simulink model "ALL_JP360_DBW_V6_5_1103"  (R2022a)
settings: Solver=FixedStepAuto  StartTime=0.0  StopTime=inf  FixedStep=0.01  RelTol=1e-3  EnableMultiTasking=on
model workspace (MAT data in the model file):
  g = 9.8
undefined symbols (not defined in the file or in its folder): canChannel, delta_v_p, IPM_Line_C0, IPM_Line_C1, IPM_Line_C2, IPM_Line_C3, M, M_p, MRR_ObjDistX, MRR_ObjDistY, MRR_ObjFusionCamID, MRR_ObjFusionSig, MRR_ObjID, MRR_ObjRelVelX, MRR_ObjRelVelY, MRR_ObjType, MRR_ObjUpdFlg, none, obj_vaild, untracktime, V, videoinput
libraries: canfdmsglib x230, canfdlib x76, slpidlib x24, simulink x18, dspstat3 x14, ctrlSharedLib x1, simulink_extras x1, imaqlib x1, realtime_pacer_lib x1, dspvision x1, visionsinks x1
(part 14 of 55)

== system ALL_JP360_DBW_V6_5_1103/MsgFromCAN/CCAN_GW_MsgFromCAN/CCAN_GW_GW_ESP_CCO_0x252 ==
  CCAN_GW_GW_ESP_CCO_0x252FromInData : Inport  OutDataTypeStr=Bus:CAN_FD_MESSAGE_BUS
  Bus Creator : BusCreator  Inputs=9  OutDataTypeStr=Bus:CCAN_GW_GW_ESP_CCO_0x252  NonVirtualBus=on
  CAN FD Unpack : canfdmsglib/CAN FD Unpack  CANdbFile=HiFire_JPT360_CCAN_Matrix_CAN_V1.72_VP_ADCU.dbc  MsgList=(none)  MsgName=GW_ESP_CCO_0x252  ProtocolMode=CAN FD  MsgIDType=Standard (11-bit identifier)  MsgIdentifier=594  MsgLength=8  SignalInfo={'Checksum_0x252','56','8','BE','unsigned','Standard','0','1','0','0','255';'ESP_CCOSts','6','2','BE','unsigned','Standard','0','1','0','0','3';'ESP_CCOTgtVel','14','5','BE','unsigned','Standard','0','1','0','0','30';'ESP_CCOWarning_Message','3','3','BE','unsigned','Standard','0','1','0','0','4';'ESP_CCO_Torque_Request','24','16','BE','unsigned','Standard','0','1','-30000','-30000','30000';'ESP_CCO_Torque_Request_Status','13','1','BE','unsigned','Standard','0','1','0','0','1';'ESP_TABSts','11','2','BE','unsigned','Standard','0','1','0','0','3';'ESP_TABWarning_Message','9','2','BE','unsigned','Standard','0','1','0','0','3';'RollingCounter_0x252','48','4','BE','unsigned','Standard','0','1','0','0','15'}  IDPort=off  TimestampPort=off  ErrorPort=off  RemotePort=off  LengthPort=off  StatusPort=off  BRSPort=off  ESIPort=off  DLCPort=off  ApplyMinMax=off
      settings: SourceProductBaseCode=XP,ME,VN  DataFormat=CANdb specified signals
  Data Type Conversion1 : DataTypeConversion  OutDataTypeStr=uint8  SaturateOnIntegerOverflow=off  RndMeth=Floor
  Data Type Conversion{2..4,7..9} (6 alike) : DataTypeConversion  OutDataTypeStr=int8  SaturateOnIntegerOverflow=off  RndMeth=Floor
  Data Type Conversion5 : DataTypeConversion  OutDataTypeStr=int16  SaturateOnIntegerOverflow=off  RndMeth=Floor
  Data Type Conversion6 : DataTypeConversion  OutDataTypeStr=boolean  SaturateOnIntegerOverflow=off  RndMeth=Floor
  CCAN_GW_GW_ESP_CCO_0x252FromOutData : Outport  OutDataTypeStr=Bus:CCAN_GW_GW_ESP_CCO_0x252
  wires:
  CAN FD Unpack/1 -> Data Type Conversion1/1
  CAN FD Unpack/2 -> Data Type Conversion2/1
  CAN FD Unpack/3 -> Data Type Conversion3/1
  CAN FD Unpack/4 -> Data Type Conversion4/1
  CAN FD Unpack/5 -> Data Type Conversion5/1
  CAN FD Unpack/6 -> Data Type Conversion6/1
  CAN FD Unpack/7 -> Data Type Conversion7/1
  CAN FD Unpack/8 -> Data Type Conversion8/1
  CAN FD Unpack/9 -> Data Type Conversion9/1
  Data Type Conversion1/1 -> Bus Creator/1  "Checksum_0x252"
  Data Type Conversion2/1 -> Bus Creator/2  "ESP_CCOSts"
  Data Type Conversion3/1 -> Bus Creator/3  "ESP_CCOTgtVel"
  Data Type Conversion4/1 -> Bus Creator/4  "ESP_CCOWarning_Message"
  Data Type Conversion5/1 -> Bus Creator/5  "ESP_CCO_Torque_Request"
  Data Type Conversion6/1 -> Bus Creator/6  "ESP_CCO_Torque_Request_Status"
  Data Type Conversion7/1 -> Bus Creator/7  "ESP_TABSts"
  Data Type Conversion8/1 -> Bus Creator/8  "ESP_TABWarning_Message"
  Data Type Conversion9/1 -> Bus Creator/9  "RollingCounter_0x252"
  Bus Creator/1 -> CCAN_GW_GW_ESP_CCO_0x252FromOutData/1  "CCAN_GW_GW_ESP_CCO_0x252FromOutData"
  CCAN_GW_GW_ESP_CCO_0x252FromInData/1 -> CAN FD Unpack/1  "CCAN_GW_GW_ESP_CCO_0x252FromInData"

== system ALL_JP360_DBW_V6_5_1103/MsgFromCAN/CCAN_GW_MsgFromCAN/CCAN_GW_IPM_0x245 ==
  CCAN_GW_IPM_0x245FromInData : Inport  OutDataTypeStr=Bus:CAN_FD_MESSAGE_BUS
  Bus Creator : BusCreator  Inputs=21  OutDataTypeStr=Bus:CCAN_GW_IPM_0x245  NonVirtualBus=on
  CAN FD Unpack : canfdmsglib/CAN FD Unpack  CANdbFile=HiFire_JPT360_CCAN_Matrix_CAN_V1.72_VP_ADCU.dbc  MsgList=(none)  MsgName=IPM_0x245  ProtocolMode=CAN FD  MsgIDType=Standard (11-bit identifier)  MsgIdentifier=581  MsgLength=8  SignalInfo={'Checksum_0x245','56','8','BE','unsigned','Standard','0','1','0','0','255';'IPM_ADAS_Alerts','43','3','BE','unsigned','Standard','0','1','0','0','7';'IPM_IHC_HighbeamReq','55','1','BE','unsigned','Standard','0','1','0','0','1';'IPM_IHC_Status','40','3','BE','unsigned','Standard','0','1','0','0','7';'IPM_LDWWarningType','52','2','BE','unsigned','Standard','0','1','0','0','3';'IPM_LaneAssitType','22','3','BE','unsigned','Standard','0','1','0','0','7';'IPM_LaneAssit_HandsonReq','54','1','BE','unsigned','Standard','0','1','0','0','1';'IPM_LaneAssit_LeftVisualization','18','2','BE','unsigned','Standard','0','1','0','0','3';'IPM_LaneAssit_RightVisualization','20','2','BE','unsigned','Standard','0','1','0','0','3';'IPM_LaneAssit_Sensitivity','16','1','BE','unsigned','Standard','0','1','0','0','1';'IPM_LaneAssit_Status','29','3','BE','unsigned','Standard','0','1','0','0','7';'IPM_LaneAssit_TorqueReq','13','11','BE','unsigned','Standard','0','0.01','-10.24','-10.24','10.22';'IPM_LaneAssit_TorqueReqStatus','10','2','BE','unsigned','Standard','0','1','0','0','3';'IPM_LaneAssit_TorqueValidity','12','1','BE','unsigned','Standard','0','1','0','0','1';'IPM_LaneAssit_WarningAudio','17','1','BE','unsigned','Standard','0','1','0','0','1';'IPM_LaneAssit_WarningVibration','9','1','BE','unsigned','Standard','0','1','0','0','1';'IPM_SLA_Spdlimit','32','8','BE','unsigned','Standard','0','1','0','0','255';'IPM_SLA_SpdlimitUnits','24','2','BE','unsigned','Standard','0','1','0','0','3';'IPM_SLA_Status','26','3','BE','unsigned','Standard','0','1','0','0','7';'IPM_TJAICA_Status','47','1','BE','unsigned','Standard','0','1','0','0','1';'RollingCounter_0x245','48','4','BE','unsigned','Standard','0','1','0','0','15'}  IDPort=off  TimestampPort=off  ErrorPort=off  RemotePort=off  LengthPort=off  StatusPort=off  BRSPort=off  ESIPort=off  DLCPort=off  ApplyMinMax=off
      settings: SourceProductBaseCode=XP,ME,VN  DataFormat=CANdb specified signals
  Data Type Conversion1 : DataTypeConversion  OutDataTypeStr=uint8  SaturateOnIntegerOverflow=off  RndMeth=Floor
  Data Type Conversion{3,7,10,14..16,20} (7 alike) : DataTypeConversion  OutDataTypeStr=boolean  SaturateOnIntegerOverflow=off  RndMeth=Floor
  Data Type Conversion{2,4..6,8..9,11,13,18..19,21} (11 alike) : DataTypeConversion  OutDataTypeStr=int8  SaturateOnIntegerOverflow=off  RndMeth=Floor
  Data Type Conversion12 : DataTypeConversion  OutDataTypeStr=single  SaturateOnIntegerOverflow=off  RndMeth=Floor
  Data Type Conversion17 : DataTypeConversion  OutDataTypeStr=uint8  SaturateOnIntegerOverflow=off  RndMeth=Floor
  CCAN_GW_IPM_0x245FromOutData : Outport  OutDataTypeStr=Bus:CCAN_GW_IPM_0x245
  wires:
  CAN FD Unpack/1 -> Data Type Conversion1/1
  CAN FD Unpack/2 -> Data Type Conversion2/1
  CAN FD Unpack/3 -> Data Type Conversion3/1
  CAN FD Unpack/4 -> Data Type Conversion4/1
  CAN FD Unpack/5 -> Data Type Conversion5/1
  CAN FD Unpack/6 -> Data Type Conversion6/1
  CAN FD Unpack/7 -> Data Type Conversion7/1
  CAN FD Unpack/8 -> Data Type Conversion8/1
  CAN FD Unpack/9 -> Data Type Conversion9/1
  CAN FD Unpack/10 -> Data Type Conversion10/1
  CAN FD Unpack/11 -> Data Type Conversion11/1
  CAN FD Unpack/12 -> Data Type Conversion12/1
  CAN FD Unpack/13 -> Data Type Conversion13/1
  CAN FD Unpack/14 -> Data Type Conversion14/1
  CAN FD Unpack/15 -> Data Type Conversion15/1
  CAN FD Unpack/16 -> Data Type Conversion16/1
  CAN FD Unpack/17 -> Data Type Conversion17/1
  CAN FD Unpack/18 -> Data Type Conversion18/1
  CAN FD Unpack/19 -> Data Type Conversion19/1
  CAN FD Unpack/20 -> Data Type Conversion20/1
  CAN FD Unpack/21 -> Data Type Conversion21/1
  Data Type Conversion1/1 -> Bus Creator/1  "Checksum_0x245"
  Data Type Conversion2/1 -> Bus Creator/2  "IPM_ADAS_Alerts"
  Data Type Conversion3/1 -> Bus Creator/3  "IPM_IHC_HighbeamReq"
  Data Type Conversion4/1 -> Bus Creator/4  "IPM_IHC_Status"
  Data Type Conversion5/1 -> Bus Creator/5  "IPM_LDWWarningType"
  Data Type Conversion6/1 -> Bus Creator/6  "IPM_LaneAssitType"
  Data Type Conversion7/1 -> Bus Creator/7  "IPM_LaneAssit_HandsonReq"
  Data Type Conversion8/1 -> Bus Creator/8  "IPM_LaneAssit_LeftVisualization"
  Data Type Conversion9/1 -> Bus Creator/9  "IPM_LaneAssit_RightVisualization"
  Data Type Conversion10/1 -> Bus Creator/10  "IPM_LaneAssit_Sensitivity"
  Data Type Conversion11/1 -> Bus Creator/11  "IPM_LaneAssit_Status"
  Data Type Conversion12/1 -> Bus Creator/12  "IPM_LaneAssit_TorqueReq"
  Data Type Conversion13/1 -> Bus Creator/13  "IPM_LaneAssit_TorqueReqStatus"
  Data Type Conversion14/1 -> Bus Creator/14  "IPM_LaneAssit_TorqueValidity"
  Data Type Conversion15/1 -> Bus Creator/15  "IPM_LaneAssit_WarningAudio"
  Data Type Conversion16/1 -> Bus Creator/16  "IPM_LaneAssit_WarningVibration"
  Data Type Conversion17/1 -> Bus Creator/17  "IPM_SLA_Spdlimit"
  Data Type Conversion18/1 -> Bus Creator/18  "IPM_SLA_SpdlimitUnits"
  Data Type Conversion19/1 -> Bus Creator/19  "IPM_SLA_Status"
  Data Type Conversion20/1 -> Bus Creator/20  "IPM_TJAICA_Status"
  Data Type Conversion21/1 -> Bus Creator/21  "RollingCounter_0x245"
  Bus Creator/1 -> CCAN_GW_IPM_0x245FromOutData/1  "CCAN_GW_IPM_0x245FromOutData"
  CCAN_GW_IPM_0x245FromInData/1 -> CAN FD Unpack/1  "CCAN_GW_IPM_0x245FromInData"

== system ALL_JP360_DBW_V6_5_1103/MsgFromCAN/CCAN_GW_MsgFromCAN/CCAN_GW_IPM_0x247 ==
  CCAN_GW_IPM_0x247FromInData : Inport  OutDataTypeStr=Bus:CAN_FD_MESSAGE_BUS
  Bus Creator : BusCreator  Inputs=7  OutDataTypeStr=Bus:CCAN_GW_IPM_0x247  NonVirtualBus=on
  CAN FD Unpack : canfdmsglib/CAN FD Unpack  CANdbFile=HiFire_JPT360_CCAN_Matrix_CAN_V1.72_VP_ADCU.dbc  MsgList=(none)  MsgName=IPM_0x247  ProtocolMode=CAN FD  MsgIDType=Standard (11-bit identifier)  MsgIdentifier=583  MsgLength=8  SignalInfo={'Checksum_0x247','56','8','BE','unsigned','Standard','0','1','0','0','255';'IPM_DCLCSts','5','3','BE','unsigned','Standard','0','1','0','0','7';'IPM_DCLC_manualfeedback','14','4','BE','unsigned','Standard','0','1','0','0','15';'IPM_ELKSts','2','3','BE','unsigned','Standard','0','1','0','0','7';'IPM_Traffic_Sign_Dis','16','8','BE','unsigned','Standard','0','1','0','0','255';'IPM_TurnIndicatorReq','12','2','BE','unsigned','Standard','0','1','0','0','3';'RollingCounter_0x247','48','4','BE','unsigned','Standard','0','1','0','0','15'}  IDPort=off  TimestampPort=off  ErrorPort=off  RemotePort=off  LengthPort=off  StatusPort=off  BRSPort=off  ESIPort=off  DLCPort=off  ApplyMinMax=off
      settings: SourceProductBaseCode=XP,ME,VN  DataFormat=CANdb specified signals
  Data Type Conversion1 : DataTypeConversion  OutDataTypeStr=uint8  SaturateOnIntegerOverflow=off  RndMeth=Floor
  Data Type Conversion{2..4,6..7} (5 alike) : DataTypeConversion  OutDataTypeStr=int8  SaturateOnIntegerOverflow=off  RndMeth=Floor
  Data Type Conversion5 : DataTypeConversion  OutDataTypeStr=uint8  SaturateOnIntegerOverflow=off  RndMeth=Floor
  CCAN_GW_IPM_0x247FromOutData : Outport  OutDataTypeStr=Bus:CCAN_GW_IPM_0x247
  wires:
  CAN FD Unpack/1 -> Data Type Conversion1/1
  CAN FD Unpack/2 -> Data Type Conversion2/1
  CAN FD Unpack/3 -> Data Type Conversion3/1
  CAN FD Unpack/4 -> Data Type Conversion4/1
  CAN FD Unpack/5 -> Data Type Conversion5/1
  CAN FD Unpack/6 -> Data Type Conversion6/1
  CAN FD Unpack/7 -> Data Type Conversion7/1
  Data Type Conversion1/1 -> Bus Creator/1  "Checksum_0x247"
  Data Type Conversion2/1 -> Bus Creator/2  "IPM_DCLCSts"
  Data Type Conversion3/1 -> Bus Creator/3  "IPM_DCLC_manualfeedback"
  Data Type Conversion4/1 -> Bus Creator/4  "IPM_ELKSts"
  Data Type Conversion5/1 -> Bus Creator/5  "IPM_Traffic_Sign_Dis"
  Data Type Conversion6/1 -> Bus Creator/6  "IPM_TurnIndicatorReq"
  Data Type Conversion7/1 -> Bus Creator/7  "RollingCounter_0x247"
  Bus Creator/1 -> CCAN_GW_IPM_0x247FromOutData/1  "CCAN_GW_IPM_0x247FromOutData"
  CCAN_GW_IPM_0x247FromInData/1 -> CAN FD Unpack/1  "CCAN_GW_IPM_0x247FromInData"

== system ALL_JP360_DBW_V6_5_1103/MsgFromCAN/CCAN_GW_MsgFromCAN/CCAN_GW_IPM_LeftLine_0x278 ==
  CCAN_GW_IPM_LeftLine_0x278FromInData : Inport  OutDataTypeStr=Bus:CAN_FD_MESSAGE_BUS
  Bus Creator : BusCreator  Inputs=6  OutDataTypeStr=Bus:CCAN_GW_IPM_LeftLine_0x278  NonVirtualBus=on
  CAN FD Unpack : canfdmsglib/CAN FD Unpack  CANdbFile=HiFire_JPT360_CCAN_Matrix_CAN_V1.72_VP_ADCU.dbc  MsgList=(none)  MsgName=IPM_LeftLine_0x278  ProtocolMode=CAN FD  MsgIDType=Standard (11-bit identifier)  MsgIdentifier=632  MsgLength=8  SignalInfo={'IPM_LedtLine_dx_start','0','8','BE','unsigned','Standard','0','0.25','0','0','63.75';'IPM_LeftLine_dx_lookhead','27','9','BE','unsigned','Standard','0','0.25','0','0','127.75';'IPM_LeftLine_dy','20','12','BE','unsigned','Standard','0','0.0039062','-8','-8','7.9961';'IPM_LeftLine_hor_curvature_alteration','58','10','BE','unsigned','Standard','0','0.0001','-0.015','-0.015','0.0873';'IPM_LeftLine_hor_curve','33','10','BE','unsigned','Standard','0','0.0001','-0.015','-0.015','0.0873';'IPM_LeftLine_yawangle','52','12','BE','unsigned','Standard','0','0.00048828','-1','-1','0.99951'}  IDPort=off  TimestampPort=off  ErrorPort=off  RemotePort=off  LengthPort=off  StatusPort=off  BRSPort=off  ESIPort=off  DLCPort=off  ApplyMinMax=off
      settings: SourceProductBaseCode=XP,ME,VN  DataFormat=CANdb specified signals
  Data Type Conversion{1..6} (6 alike) : DataTypeConversion  OutDataTypeStr=single  SaturateOnIntegerOverflow=off  RndMeth=Floor
  CCAN_GW_IPM_LeftLine_0x278FromOutData : Outport  OutDataTypeStr=Bus:CCAN_GW_IPM_LeftLine_0x278
  wires:
  CAN FD Unpack/1 -> Data Type Conversion1/1
  CAN FD Unpack/2 -> Data Type Conversion2/1
  CAN FD Unpack/3 -> Data Type Conversion3/1
  CAN FD Unpack/4 -> Data Type Conversion4/1
  CAN FD Unpack/5 -> Data Type Conversion5/1
  CAN FD Unpack/6 -> Data Type Conversion6/1
  Data Type Conversion1/1 -> Bus Creator/1  "IPM_LedtLine_dx_start"
  Data Type Conversion2/1 -> Bus Creator/2  "IPM_LeftLine_dx_lookhead"
  Data Type Conversion3/1 -> Bus Creator/3  "IPM_LeftLine_dy"
  Data Type Conversion4/1 -> Bus Creator/4  "IPM_LeftLine_hor_curvature_alteration"
  Data Type Conversion5/1 -> Bus Creator/5  "IPM_LeftLine_hor_curve"
  Data Type Conversion6/1 -> Bus Creator/6  "IPM_LeftLine_yawangle"
  Bus Creator/1 -> CCAN_GW_IPM_LeftLine_0x278FromOutData/1  "CCAN_GW_IPM_LeftLine_0x278FromOutData"
  CCAN_GW_IPM_LeftLine_0x278FromInData/1 -> CAN FD Unpack/1  "CCAN_GW_IPM_LeftLine_0x278FromInData"

== system ALL_JP360_DBW_V6_5_1103/MsgFromCAN/CCAN_GW_MsgFromCAN/CCAN_GW_IPM_LeftLine_0x280 ==
  CCAN_GW_IPM_LeftLine_0x280FromInData : Inport  OutDataTypeStr=Bus:CAN_FD_MESSAGE_BUS
  Bus Creator : BusCreator  Inputs=9  OutDataTypeStr=Bus:CCAN_GW_IPM_LeftLine_0x280  NonVirtualBus=on
  CAN FD Unpack : canfdmsglib/CAN FD Unpack  CANdbFile=HiFire_JPT360_CCAN_Matrix_CAN_V1.72_VP_ADCU.dbc  MsgList=(none)  MsgName=IPM_LeftLine_0x280  ProtocolMode=CAN FD  MsgIDType=Standard (11-bit identifier)  MsgIdentifier=640  MsgLength=8  SignalInfo={'IPM_LaneAssit_LeftLeftVisualization','0','2','BE','unsigned','Standard','0','1','0','0','3';'IPM_LeftLeftLine_Color','13','3','BE','unsigned','Standard','0','1','0','0','7';'IPM_LeftLeftLine_Type','10','3','BE','unsigned','Standard','0','1','0','0','7';'IPM_LeftLeftLine_curvature_alteration','56','12','BE','unsigned','Standard','0','0.0001','-0.015','-0.015','0.0873';'IPM_LeftLeftLine_dy','28','12','BE','unsigned','Standard','0','0.0039062','-8','-8','7.9961';'IPM_LeftLeftLine_hor_curve','33','10','BE','unsigned','Standard','0','0.0001','-0.015','-0.015','0.0873';'IPM_LeftLeftLine_yawangle','52','12','BE','unsigned','Standard','0','0.00048828','-1','-1','0.99951';'IPM_LeftLine_Color','5','3','BE','unsigned','Standard','0','1','0','0','7';'IPM_LeftLine_Type','2','3','BE','unsigned','Standard','0','1','0','0','7'}  IDPort=off  TimestampPort=off  ErrorPort=off  RemotePort=off  LengthPort=off  StatusPort=off  BRSPort=off  ESIPort=off  DLCPort=off  ApplyMinMax=off
      settings: SourceProductBaseCode=XP,ME,VN  DataFormat=CANdb specified signals
  Data Type Conversion{1..3,8..9} (5 alike) : DataTypeConversion  OutDataTypeStr=int8  SaturateOnIntegerOverflow=off  RndMeth=Floor
  Data Type Conversion{4..7} (4 alike) : DataTypeConversion  OutDataTypeStr=single  SaturateOnIntegerOverflow=off  RndMeth=Floor
  CCAN_GW_IPM_LeftLine_0x280FromOutData : Outport  OutDataTypeStr=Bus:CCAN_GW_IPM_LeftLine_0x280
  wires:
  CAN FD Unpack/1 -> Data Type Conversion1/1
  CAN FD Unpack/2 -> Data Type Conversion2/1
  CAN FD Unpack/3 -> Data Type Conversion3/1
  CAN FD Unpack/4 -> Data Type Conversion4/1
  CAN FD Unpack/5 -> Data Type Conversion5/1
  CAN FD Unpack/6 -> Data Type Conversion6/1
  CAN FD Unpack/7 -> Data Type Conversion7/1
  CAN FD Unpack/8 -> Data Type Conversion8/1
  CAN FD Unpack/9 -> Data Type Conversion9/1
  Data Type Conversion1/1 -> Bus Creator/1  "IPM_LaneAssit_LeftLeftVisualization"
  Data Type Conversion2/1 -> Bus Creator/2  "IPM_LeftLeftLine_Color"
  Data Type Conversion3/1 -> Bus Creator/3  "IPM_LeftLeftLine_Type"
  Data Type Conversion4/1 -> Bus Creator/4  "IPM_LeftLeftLine_curvature_alteration"
  Data Type Conversion5/1 -> Bus Creator/5  "IPM_LeftLeftLine_dy"
  Data Type Conversion6/1 -> Bus Creator/6  "IPM_LeftLeftLine_hor_curve"
  Data Type Conversion7/1 -> Bus Creator/7  "IPM_LeftLeftLine_yawangle"
  Data Type Conversion8/1 -> Bus Creator/8  "IPM_LeftLine_Color"
  Data Type Conversion9/1 -> Bus Creator/9  "IPM_LeftLine_Type"
  Bus Creator/1 -> CCAN_GW_IPM_LeftLine_0x280FromOutData/1  "CCAN_GW_IPM_LeftLine_0x280FromOutData"
  CCAN_GW_IPM_LeftLine_0x280FromInData/1 -> CAN FD Unpack/1  "CCAN_GW_IPM_LeftLine_0x280FromInData"

== system ALL_JP360_DBW_V6_5_1103/MsgFromCAN/CCAN_GW_MsgFromCAN/CCAN_GW_IPM_RightLine_0x490 ==
  CCAN_GW_IPM_RightLine_0x490FromInData : Inport  OutDataTypeStr=Bus:CAN_FD_MESSAGE_BUS
  Bus Creator : BusCreator  Inputs=6  OutDataTypeStr=Bus:CCAN_GW_IPM_RightLine_0x490  NonVirtualBus=on
  CAN FD Unpack : canfdmsglib/CAN FD Unpack  CANdbFile=HiFire_JPT360_CCAN_Matrix_CAN_V1.72_VP_ADCU.dbc  MsgList=(none)  MsgName=IPM_RightLine_0x490  ProtocolMode=CAN FD  MsgIDType=Standard (11-bit identifier)  MsgIdentifier=1168  MsgLength=8  SignalInfo={'IPM_RightLine_dx_lookhead','27','9','BE','unsigned','Standard','0','0.25','0','0','127.75';'IPM_RightLine_dx_start','0','8','BE','unsigned','Standard','0','0.25','0','0','63.75';'IPM_RightLine_dy','20','12','BE','unsigned','Standard','0','0.0039062','-8','-8','7.9961';'IPM_RightLine_hor_curvature_alteration','58','10','BE','unsigned','Standard','0','0.0001','-0.015','-0.015','0.0873';'IPM_RightLine_hor_curve','33','10','BE','unsigned','Standard','0','0.0001','-0.015','-0.015','0.0873';'IPM_RightLine_yawangle','52','12','BE','unsigned','Standard','0','0.00048828','-1','-1','0.99951'}  IDPort=off  TimestampPort=off  ErrorPort=off  RemotePort=off  LengthPort=off  StatusPort=off  BRSPort=off  ESIPort=off  DLCPort=off  ApplyMinMax=off
      settings: SourceProductBaseCode=XP,ME,VN  DataFormat=CANdb specified signals
  Data Type Conversion{1..6} (6 alike) : DataTypeConversion  OutDataTypeStr=single  SaturateOnIntegerOverflow=off  RndMeth=Floor
  CCAN_GW_IPM_RightLine_0x490FromOutData : Outport  OutDataTypeStr=Bus:CCAN_GW_IPM_RightLine_0x490
  wires:
  CAN FD Unpack/1 -> Data Type Conversion1/1
  CAN FD Unpack/2 -> Data Type Conversion2/1
  CAN FD Unpack/3 -> Data Type Conversion3/1
  CAN FD Unpack/4 -> Data Type Conversion4/1
  CAN FD Unpack/5 -> Data Type Conversion5/1
  CAN FD Unpack/6 -> Data Type Conversion6/1
  Data Type Conversion1/1 -> Bus Creator/1  "IPM_RightLine_dx_lookhead"
  Data Type Conversion2/1 -> Bus Creator/2  "IPM_RightLine_dx_start"
  Data Type Conversion3/1 -> Bus Creator/3  "IPM_RightLine_dy"
  Data Type Conversion4/1 -> Bus Creator/4  "IPM_RightLine_hor_curvature_alteration"
  Data Type Conversion5/1 -> Bus Creator/5  "IPM_RightLine_hor_curve"
  Data Type Conversion6/1 -> Bus Creator/6  "IPM_RightLine_yawangle"
  Bus Creator/1 -> CCAN_GW_IPM_RightLine_0x490FromOutData/1  "CCAN_GW_IPM_RightLine_0x490FromOutData"
  CCAN_GW_IPM_RightLine_0x490FromInData/1 -> CAN FD Unpack/1  "CCAN_GW_IPM_RightLine_0x490FromInData"

== system ALL_JP360_DBW_V6_5_1103/MsgFromCAN/CCAN_GW_MsgFromCAN/CCAN_GW_IPM_RightLine_0x491 ==
  CCAN_GW_IPM_RightLine_0x491FromInData : Inport  OutDataTypeStr=Bus:CAN_FD_MESSAGE_BUS
  Bus Creator : BusCreator  Inputs=9  OutDataTypeStr=Bus:CCAN_GW_IPM_RightLine_0x491  NonVirtualBus=on
  CAN FD Unpack : canfdmsglib/CAN FD Unpack  CANdbFile=HiFire_JPT360_CCAN_Matrix_CAN_V1.72_VP_ADCU.dbc  MsgList=(none)  MsgName=IPM_RightLine_0x491  ProtocolMode=CAN FD  MsgIDType=Standard (11-bit identifier)  MsgIdentifier=1169  MsgLength=8  SignalInfo={'IPM_LaneAssit_RightRightVisualization','0','2','BE','unsigned','Standard','0','1','0','0','3';'IPM_RighRightLine_Color','13','3','BE','unsigned','Standard','0','1','0','0','7';'IPM_RightLine_Color','5','3','BE','unsigned','Standard','0','1','0','0','7';'IPM_RightLine_Type','2','3','BE','unsigned','Standard','0','1','0','0','7';'IPM_RightRighLine_Type','10','3','BE','unsigned','Standard','0','1','0','0','7';'IPM_RightRightLine_curvature_alteration','56','12','BE','unsigned','Standard','0','0.0001','-0.015','-0.015','0.0873';'IPM_RightRightLine_dy','28','12','BE','unsigned','Standard','0','0.0039062','-8','-8','7.9961';'IPM_RightRightLine_hor_curve','33','10','BE','unsigned','Standard','0','0.0001','-0.015','-0.015','0.0873';'IPM_RightRightLine_yawangle','52','12','BE','unsigned','Standard','0','0.00048828','-1','-1','0.99951'}  IDPort=off  TimestampPort=off  ErrorPort=off  RemotePort=off  LengthPort=off  StatusPort=off  BRSPort=off  ESIPort=off  DLCPort=off  ApplyMinMax=off
      settings: SourceProductBaseCode=XP,ME,VN  DataFormat=CANdb specified signals
  Data Type Conversion{1..5} (5 alike) : DataTypeConversion  OutDataTypeStr=int8  SaturateOnIntegerOverflow=off  RndMeth=Floor
  Data Type Conversion{6..9} (4 alike) : DataTypeConversion  OutDataTypeStr=single  SaturateOnIntegerOverflow=off  RndMeth=Floor
  CCAN_GW_IPM_RightLine_0x491FromOutData : Outport  OutDataTypeStr=Bus:CCAN_GW_IPM_RightLine_0x491
  wires:
  CAN FD Unpack/1 -> Data Type Conversion1/1
  CAN FD Unpack/2 -> Data Type Conversion2/1
  CAN FD Unpack/3 -> Data Type Conversion3/1
  CAN FD Unpack/4 -> Data Type Conversion4/1
  CAN FD Unpack/5 -> Data Type Conversion5/1
  CAN FD Unpack/6 -> Data Type Conversion6/1
  CAN FD Unpack/7 -> Data Type Conversion7/1
  CAN FD Unpack/8 -> Data Type Conversion8/1
  CAN FD Unpack/9 -> Data Type Conversion9/1
  Data Type Conversion1/1 -> Bus Creator/1  "IPM_LaneAssit_RightRightVisualization"
  Data Type Conversion2/1 -> Bus Creator/2  "IPM_RighRightLine_Color"
  Data Type Conversion3/1 -> Bus Creator/3  "IPM_RightLine_Color"
  Data Type Conversion4/1 -> Bus Creator/4  "IPM_RightLine_Type"
  Data Type Conversion5/1 -> Bus Creator/5  "IPM_RightRighLine_Type"
  Data Type Conversion6/1 -> Bus Creator/6  "IPM_RightRightLine_curvature_alteration"
  Data Type Conversion7/1 -> Bus Creator/7  "IPM_RightRightLine_dy"
  Data Type Conversion8/1 -> Bus Creator/8  "IPM_RightRightLine_hor_curve"
  Data Type Conversion9/1 -> Bus Creator/9  "IPM_RightRightLine_yawangle"
  Bus Creator/1 -> CCAN_GW_IPM_RightLine_0x491FromOutData/1  "CCAN_GW_IPM_RightLine_0x491FromOutData"
  CCAN_GW_IPM_RightLine_0x491FromInData/1 -> CAN FD Unpack/1  "CCAN_GW_IPM_RightLine_0x491FromInData"

== system ALL_JP360_DBW_V6_5_1103/MsgFromCAN/CCAN_GW_MsgFromCAN/CCAN_GW_IPM_VLC_0x293 ==
  CCAN_GW_IPM_VLC_0x293FromInData : Inport  OutDataTypeStr=Bus:CAN_FD_MESSAGE_BUS
  Bus Creator : BusCreator  Inputs=4  OutDataTypeStr=Bus:CCAN_GW_IPM_VLC_0x293  NonVirtualBus=on
  CAN FD Unpack : canfdmsglib/CAN FD Unpack  CANdbFile=HiFire_JPT360_CCAN_Matrix_CAN_V1.72_VP_ADCU.dbc  MsgList=(none)  MsgName=IPM_VLC_0x293  ProtocolMode=CAN FD  MsgIDType=Standard (11-bit identifier)  MsgIdentifier=659  MsgLength=8  SignalInfo={'ACC_Torque_Request','16','16','BE','unsigned','Standard','0','0.5','-15000','-15000','15000';'ACC_Torque_Request_Status','7','1','BE','unsigned','Standard','0','1','0','0','1';'Checksum_0x293','56','8','BE','unsigned','Standard','0','1','0','0','255';'RollingCounter_0x293','48','4','BE','unsigned','Standard','0','1','0','0','15'}  IDPort=off  TimestampPort=off  ErrorPort=off  RemotePort=off  LengthPort=off  StatusPort=off  BRSPort=off  ESIPort=off  DLCPort=off  ApplyMinMax=off
      settings: SourceProductBaseCode=XP,ME,VN  DataFormat=CANdb specified signals
  Data Type Conversion1 : DataTypeConversion  OutDataTypeStr=single  SaturateOnIntegerOverflow=off  RndMeth=Floor
  Data Type Conversion2 : DataTypeConversion  OutDataTypeStr=boolean  SaturateOnIntegerOverflow=off  RndMeth=Floor
  Data Type Conversion3 : DataTypeConversion  OutDataTypeStr=uint8  SaturateOnIntegerOverflow=off  RndMeth=Floor
  Data Type Conversion4 : DataTypeConversion  OutDataTypeStr=int8  SaturateOnIntegerOverflow=off  RndMeth=Floor
  CCAN_GW_IPM_VLC_0x293FromOutData : Outport  OutDataTypeStr=Bus:CCAN_GW_IPM_VLC_0x293
  wires:
  CAN FD Unpack/1 -> Data Type Conversion1/1
  CAN FD Unpack/2 -> Data Type Conversion2/1
  CAN FD Unpack/3 -> Data Type Conversion3/1
  CAN FD Unpack/4 -> Data Type Conversion4/1
  Data Type Conversion1/1 -> Bus Creator/1  "ACC_Torque_Request"
  Data Type Conversion2/1 -> Bus Creator/2  "ACC_Torque_Request_Status"
  Data Type Conversion3/1 -> Bus Creator/3  "Checksum_0x293"
  Data Type Conversion4/1 -> Bus Creator/4  "RollingCounter_0x293"
  Bus Creator/1 -> CCAN_GW_IPM_VLC_0x293FromOutData/1  "CCAN_GW_IPM_VLC_0x293FromOutData"
  CCAN_GW_IPM_VLC_0x293FromInData/1 -> CAN FD Unpack/1  "CCAN_GW_IPM_VLC_0x293FromInData"

== system ALL_JP360_DBW_V6_5_1103/MsgFromCAN/CCAN_GW_MsgFromCAN/CCAN_GW_MRR_0x238 ==
  CCAN_GW_MRR_0x238FromInData : Inport  OutDataTypeStr=Bus:CAN_FD_MESSAGE_BUS
  Bus Creator : BusCreator  Inputs=7  OutDataTypeStr=Bus:CCAN_GW_MRR_0x238  NonVirtualBus=on
  CAN FD Unpack : canfdmsglib/CAN FD Unpack  CANdbFile=HiFire_JPT360_CCAN_Matrix_CAN_V1.72_VP_ADCU.dbc  MsgList=(none)  MsgName=MRR_0x238  ProtocolMode=CAN FD  MsgIDType=Standard (11-bit identifier)  MsgIdentifier=568  MsgLength=8  SignalInfo={'ACC_TgtAx','53','11','BE','unsigned','Standard','0','0.05','-5','-5','7.75';'ACC_TgtAxLowerComftBand','8','8','BE','unsigned','Standard','0','0.05','0','0','3.2';'ACC_TgtAxLowerLim','24','8','BE','unsigned','Standard','0','0.1','-12.7','-12.7','0';'ACC_TgtAxUpperComftBand','0','8','BE','unsigned','Standard','0','0.05','0','0','3.2';'ACC_TgtAxUpperLim','16','8','BE','unsigned','Standard','0','0.1','0','0','12.7';'Checksum_0x238','56','8','BE','unsigned','Standard','0','1','0','0','255';'RollingCounter_0x238','48','4','BE','unsigned','Standard','0','1','0','0','15'}  IDPort=off  TimestampPort=off  ErrorPort=off  RemotePort=off  LengthPort=off  StatusPort=off  BRSPort=off  ESIPort=off  DLCPort=off  ApplyMinMax=off
      settings: SourceProductBaseCode=XP,ME,VN  DataFormat=CANdb specified signals
  Data Type Conversion{1..5} (5 alike) : DataTypeConversion  OutDataTypeStr=single  SaturateOnIntegerOverflow=off  RndMeth=Floor
  Data Type Conversion6 : DataTypeConversion  OutDataTypeStr=uint8  SaturateOnIntegerOverflow=off  RndMeth=Floor
  Data Type Conversion7 : DataTypeConversion  OutDataTypeStr=int8  SaturateOnIntegerOverflow=off  RndMeth=Floor
  CCAN_GW_MRR_0x238FromOutData : Outport  OutDataTypeStr=Bus:CCAN_GW_MRR_0x238
  wires:
  CAN FD Unpack/1 -> Data Type Conversion1/1
  CAN FD Unpack/2 -> Data Type Conversion2/1
  CAN FD Unpack/3 -> Data Type Conversion3/1
  CAN FD Unpack/4 -> Data Type Conversion4/1
  CAN FD Unpack/5 -> Data Type Conversion5/1
  CAN FD Unpack/6 -> Data Type Conversion6/1
  CAN FD Unpack/7 -> Data Type Conversion7/1
  Data Type Conversion1/1 -> Bus Creator/1  "ACC_TgtAx"
  Data Type Conversion2/1 -> Bus Creator/2  "ACC_TgtAxLowerComftBand"
  Data Type Conversion3/1 -> Bus Creator/3  "ACC_TgtAxLowerLim"
  Data Type Conversion4/1 -> Bus Creator/4  "ACC_TgtAxUpperComftBand"
  Data Type Conversion5/1 -> Bus Creator/5  "ACC_TgtAxUpperLim"
  Data Type Conversion6/1 -> Bus Creator/6  "Checksum_0x238"
  Data Type Conversion7/1 -> Bus Creator/7  "RollingCounter_0x238"
  Bus Creator/1 -> CCAN_GW_MRR_0x238FromOutData/1  "CCAN_GW_MRR_0x238FromOutData"
  CCAN_GW_MRR_0x238FromInData/1 -> CAN FD Unpack/1  "CCAN_GW_MRR_0x238FromInData"

== system ALL_JP360_DBW_V6_5_1103/MsgFromCAN/CCAN_GW_MsgFromCAN/CCAN_GW_MRR_0x239 ==
  CCAN_GW_MRR_0x239FromInData : Inport  OutDataTypeStr=Bus:CAN_FD_MESSAGE_BUS
  Bus Creator : BusCreator  Inputs=16  OutDataTypeStr=Bus:CCAN_GW_MRR_0x239  NonVirtualBus=on
  CAN FD Unpack : canfdmsglib/CAN FD Unpack  CANdbFile=HiFire_JPT360_CCAN_Matrix_CAN_V1.72_VP_ADCU.dbc  MsgList=(none)  MsgName=MRR_0x239  ProtocolMode=CAN FD  MsgIDType=Standard (11-bit identifier)  MsgIdentifier=569  MsgLength=8  SignalInfo={'ABA_Level','8','2','BE','unsigned','Standard','0','1','0','0','3';'ABA_Req','23','1','BE','unsigned','Standard','0','1','0','0','1';'ABP_Req','21','1','BE','unsigned','Standard','0','1','0','0','1';'ACC_BrakePreferred','1','1','BE','unsigned','Standard','0','1','0','0','1';'ACC_DriveOff','15','1','BE','unsigned','Standard','0','1','0','0','1';'ACC_StandstillReq','14','1','BE','unsigned','Standard','0','1','0','0','1';'ACC_Status','3','3','BE','unsigned','Standard','0','1','0','0','7';'ACC_VLCMinBrakingReq','0','1','BE','unsigned','Standard','0','1','0','0','1';'ACC_VLCShutdownMode','6','2','BE','unsigned','Standard','0','1','0','0','3';'AEB_Req','13','1','BE','unsigned','Standard','0','1','0','0','1';'AEB_TgtAx','32','16','BE','unsigned','Standard','0','0.05','-16','-16','16';'AWB_Level','16','4','BE','unsigned','Standard','0','1','0','0','15';'AWB_Req','22','1','BE','unsigned','Standard','0','1','0','0','1';'Checksum_0x239','56','8','BE','unsigned','Standard','0','1','0','0','255';'EBA_Req','12','1','BE','unsigned','Standard','0','1','0','0','1';'RollingCounter_0x239','48','4','BE','unsigned','Standard','0','1','0','0','15'}  IDPort=off  TimestampPort=off  ErrorPort=off  RemotePort=off  LengthPort=off  StatusPort=off  BRSPort=off  ESIPort=off  DLCPort=off  ApplyMinMax=off
      settings: SourceProductBaseCode=XP,ME,VN  DataFormat=CANdb specified signals
  Data Type Conversion{1,7,9,12,16} (5 alike) : DataTypeConversion  OutDataTypeStr=int8  SaturateOnIntegerOverflow=off  RndMeth=Floor
  Data Type Conversion{2..6,8,10,13,15} (9 alike) : DataTypeConversion  OutDataTypeStr=boolean  SaturateOnIntegerOverflow=off  RndMeth=Floor
  Data Type Conversion11 : DataTypeConversion  OutDataTypeStr=single  SaturateOnIntegerOverflow=off  RndMeth=Floor
  Data Type Conversion14 : DataTypeConversion  OutDataTypeStr=uint8  SaturateOnIntegerOverflow=off  RndMeth=Floor
  CCAN_GW_MRR_0x239FromOutData : Outport  OutDataTypeStr=Bus:CCAN_GW_MRR_0x239
  wires:
  CAN FD Unpack/1 -> Data Type Conversion1/1
  CAN FD Unpack/2 -> Data Type Conversion2/1
  CAN FD Unpack/3 -> Data Type Conversion3/1
  CAN FD Unpack/4 -> Data Type Conversion4/1
  CAN FD Unpack/5 -> Data Type Conversion5/1
  CAN FD Unpack/6 -> Data Type Conversion6/1
  CAN FD Unpack/7 -> Data Type Conversion7/1
  CAN FD Unpack/8 -> Data Type Conversion8/1
  CAN FD Unpack/9 -> Data Type Conversion9/1
  CAN FD Unpack/10 -> Data Type Conversion10/1
  CAN FD Unpack/11 -> Data Type Conversion11/1
  CAN FD Unpack/12 -> Data Type Conversion12/1
  CAN FD Unpack/13 -> Data Type Conversion13/1
  CAN FD Unpack/14 -> Data Type Conversion14/1
  CAN FD Unpack/15 -> Data Type Conversion15/1
  CAN FD Unpack/16 -> Data Type Conversion16/1
  Data Type Conversion1/1 -> Bus Creator/1  "ABA_Level"
  Data Type Conversion2/1 -> Bus Creator/2  "ABA_Req"
  Data Type Conversion3/1 -> Bus Creator/3  "ABP_Req"
  Data Type Conversion4/1 -> Bus Creator/4  "ACC_BrakePreferred"
  Data Type Conversion5/1 -> Bus Creator/5  "ACC_DriveOff"
  Data Type Conversion6/1 -> Bus Creator/6  "ACC_StandstillReq"
  Data Type Conversion7/1 -> Bus Creator/7  "ACC_Status"
  Data Type Conversion8/1 -> Bus Creator/8  "ACC_VLCMinBrakingReq"
  Data Type Conversion9/1 -> Bus Creator/9  "ACC_VLCShutdownMode"
  Data Type Conversion10/1 -> Bus Creator/10  "AEB_Req"
  Data Type Conversion11/1 -> Bus Creator/11  "AEB_TgtAx"
  Data Type Conversion12/1 -> Bus Creator/12  "AWB_Level"
  Data Type Conversion13/1 -> Bus Creator/13  "AWB_Req"
  Data Type Conversion14/1 -> Bus Creator/14  "Checksum_0x239"
  Data Type Conversion15/1 -> Bus Creator/15  "EBA_Req"
  Data Type Conversion16/1 -> Bus Creator/16  "RollingCounter_0x239"
  Bus Creator/1 -> CCAN_GW_MRR_0x239FromOutData/1  "CCAN_GW_MRR_0x239FromOutData"
  CCAN_GW_MRR_0x239FromInData/1 -> CAN FD Unpack/1  "CCAN_GW_MRR_0x239FromInData"

== system ALL_JP360_DBW_V6_5_1103/MsgFromCAN/CCAN_GW_MsgFromCAN/CCAN_GW_MRR_0x246 ==
  CCAN_GW_MRR_0x246FromInData : Inport  OutDataTypeStr=Bus:CAN_FD_MESSAGE_BUS
  Bus Creator : BusCreator  Inputs=19  OutDataTypeStr=Bus:CCAN_GW_MRR_0x246  NonVirtualBus=on
  CAN FD Unpack : canfdmsglib/CAN FD Unpack  CANdbFile=HiFire_JPT360_CCAN_Matrix_CAN_V1.72_VP_ADCU.dbc  MsgList=(none)  MsgName=MRR_0x246  ProtocolMode=CAN FD  MsgIDType=Standard (11-bit identifier)  MsgIdentifier=582  MsgLength=8  SignalInfo={'ACC_EngineStartstop','28','2','BE','unsigned','Standard','0','1','0','0','3';'ACC_FailInfo','19','1','BE','unsigned','Standard','0','1','0','0','1';'ACC_ModeHMI','16','3','BE','unsigned','Standard','0','1','0','0','7';'ACC_ObjDetected','8','1','BE','unsigned','Standard','0','1','0','0','1';'ACC_SpdSetValue','15','9','BE','unsigned','Standard','0','0.5','0','0','255.5';'ACC_TakeOverReq','20','1','BE','unsigned','Standard','0','1','0','0','1';'ACC_TarObjBarDis','12','3','BE','unsigned','Standard','0','1','0','0','7';'ACC_Textinfo','52','6','BE','unsigned','Standard','0','1','0','0','63';'ACC_TimeGapSet','9','3','BE','unsigned','Standard','0','1','0','0','7';'AEB_Status','25','3','BE','unsigned','Standard','0','1','0','0','7';'Checksum_0x246','56','8','BE','unsigned','Standard','0','1','0','0','255';'FCW_PedWarningLevel1','21','1','BE','unsigned','Standard','0','1','0','0','1';'FCW_PedWarningLevel2','24','1','BE','unsigned','Standard','0','1','0','0','1';'FCW_Sensitive','22','2','BE','unsigned','Standard','0','1','0','0','3';'FCW_Status','37','3','BE','unsigned','Standard','0','1','0','0','7';'FCW_WarningLevel1','31','1','BE','unsigned','Standard','0','1','0','0','1';'FCW_WarningLevel2','30','1','BE','unsigned','Standard','0','1','0','0','1';'Obj_Speed','42','8','BE','unsigned','Standard','0','1','0','0','255';'RollingCounter_0x246','48','4','BE','unsigned','Standard','0','1','0','0','15'}  IDPort=off  TimestampPort=off  ErrorPort=off  RemotePort=off  LengthPort=off  StatusPort=off  BRSPort=off  ESIPort=off  DLCPort=off  ApplyMinMax=off
      settings: SourceProductBaseCode=XP,ME,VN  DataFormat=CANdb specified signals
  Data Type Conversion{1,3,7..10,14..15,19} (9 alike) : DataTypeConversion  OutDataTypeStr=int8  SaturateOnIntegerOverflow=off  RndMeth=Floor
  Data Type Conversion11 : DataTypeConversion  OutDataTypeStr=uint8  SaturateOnIntegerOverflow=off  RndMeth=Floor
  Data Type Conversion{2,4,6,12..13,16..17} (7 alike) : DataTypeConversion  OutDataTypeStr=boolean  SaturateOnIntegerOverflow=off  RndMeth=Floor
  Data Type Conversion18 : DataTypeConversion  OutDataTypeStr=uint8  SaturateOnIntegerOverflow=off  RndMeth=Floor
  Data Type Conversion5 : DataTypeConversion  OutDataTypeStr=single  SaturateOnIntegerOverflow=off  RndMeth=Floor
  CCAN_GW_MRR_0x246FromOutData : Outport  OutDataTypeStr=Bus:CCAN_GW_MRR_0x246
  wires:
  CAN FD Unpack/1 -> Data Type Conversion1/1
  CAN FD Unpack/2 -> Data Type Conversion2/1
  CAN FD Unpack/3 -> Data Type Conversion3/1
  CAN FD Unpack/4 -> Data Type Conversion4/1
  CAN FD Unpack/5 -> Data Type Conversion5/1
  CAN FD Unpack/6 -> Data Type Conversion6/1
  CAN FD Unpack/7 -> Data Type Conversion7/1
  CAN FD Unpack/8 -> Data Type Conversion8/1
  CAN FD Unpack/9 -> Data Type Conversion9/1
  CAN FD Unpack/10 -> Data Type Conversion10/1
  CAN FD Unpack/11 -> Data Type Conversion11/1
  CAN FD Unpack/12 -> Data Type Conversion12/1
  CAN FD Unpack/13 -> Data Type Conversion13/1
  CAN FD Unpack/14 -> Data Type Conversion14/1
  CAN FD Unpack/15 -> Data Type Conversion15/1
  CAN FD Unpack/16 -> Data Type Conversion16/1
  CAN FD Unpack/17 -> Data Type Conversion17/1
  CAN FD Unpack/18 -> Data Type Conversion18/1
  CAN FD Unpack/19 -> Data Type Conversion19/1
  Data Type Conversion1/1 -> Bus Creator/1  "ACC_EngineStartstop"
  Data Type Conversion2/1 -> Bus Creator/2  "ACC_FailInfo"
  Data Type Conversion3/1 -> Bus Creator/3  "ACC_ModeHMI"
  Data Type Conversion4/1 -> Bus Creator/4  "ACC_ObjDetected"
  Data Type Conversion5/1 -> Bus Creator/5  "ACC_SpdSetValue"
  Data Type Conversion6/1 -> Bus Creator/6  "ACC_TakeOverReq"
  Data Type Conversion7/1 -> Bus Creator/7  "ACC_TarObjBarDis"
  Data Type Conversion8/1 -> Bus Creator/8  "ACC_Textinfo"
  Data Type Conversion9/1 -> Bus Creator/9  "ACC_TimeGapSet"
  Data Type Conversion10/1 -> Bus Creator/10  "AEB_Status"
  Data Type Conversion11/1 -> Bus Creator/11  "Checksum_0x246"
  Data Type Conversion12/1 -> Bus Creator/12  "FCW_PedWarningLevel1"
  Data Type Conversion13/1 -> Bus Creator/13  "FCW_PedWarningLevel2"
  Data Type Conversion14/1 -> Bus Creator/14  "FCW_Sensitive"
  Data Type Conversion15/1 -> Bus Creator/15  "FCW_Status"
  Data Type Conversion16/1 -> Bus Creator/16  "FCW_WarningLevel1"
  Data Type Conversion17/1 -> Bus Creator/17  "FCW_WarningLevel2"
  Data Type Conversion18/1 -> Bus Creator/18  "Obj_Speed"
  Data Type Conversion19/1 -> Bus Creator/19  "RollingCounter_0x246"
  Bus Creator/1 -> CCAN_GW_MRR_0x246FromOutData/1  "CCAN_GW_MRR_0x246FromOutData"
  CCAN_GW_MRR_0x246FromInData/1 -> CAN FD Unpack/1  "CCAN_GW_MRR_0x246FromInData"

== system ALL_JP360_DBW_V6_5_1103/MsgFromCAN/CCAN_GW_MsgFromCAN/CCAN_GW_MRR_FRObj_0x279 ==
  CCAN_GW_MRR_FRObj_0x279FromInData : Inport  OutDataTypeStr=Bus:CAN_FD_MESSAGE_BUS
  Bus Creator : BusCreator  Inputs=8  OutDataTypeStr=Bus:CCAN_GW_MRR_FRObj_0x279  NonVirtualBus=on
  CAN FD Unpack : canfdmsglib/CAN FD Unpack  CANdbFile=HiFire_JPT360_CCAN_Matrix_CAN_V1.72_VP_ADCU.dbc  MsgList=(none)  MsgName=MRR_FRObj_0x279  ProtocolMode=CAN FD  MsgIDType=Standard (11-bit identifier)  MsgIdentifier=633  MsgLength=8  SignalInfo={'MRR_FFTargetDetection','54','1','BE','unsigned','Standard','0','1','0','0','1';'MRR_FF_Obj_0x_class','40','3','BE','unsigned','Standard','0','1','0','0','7';'MRR_FF_Object_dx','36','12','BE','unsigned','Standard','0','0.0625','0','0','255.875';'MRR_FF_Object_dy','43','9','BE','unsigned','Standard','0','0.0625','-15','-15','15';'MRR_F_Obj_0x_class','16','3','BE','unsigned','Standard','0','1','0','0','7';'MRR_F_Object_dx','12','12','BE','unsigned','Standard','0','0.0625','0','0','255.875';'MRR_F_Object_dy','19','9','BE','unsigned','Standard','0','0.0625','-15','-15','15';'MRR_PedDetection','55','1','BE','unsigned','Standard','0','1','0','0','1'}  IDPort=off  TimestampPort=off  ErrorPort=off  RemotePort=off  LengthPort=off  StatusPort=off  BRSPort=off  ESIPort=off  DLCPort=off  ApplyMinMax=off
      settings: SourceProductBaseCode=XP,ME,VN  DataFormat=CANdb specified signals
  Data Type Conversion1 : DataTypeConversion  OutDataTypeStr=boolean  SaturateOnIntegerOverflow=off  RndMeth=Floor
  Data Type Conversion2 : DataTypeConversion  OutDataTypeStr=int8  SaturateOnIntegerOverflow=off  RndMeth=Floor
  Data Type Conversion{3..4,6..7} (4 alike) : DataTypeConversion  OutDataTypeStr=single  SaturateOnIntegerOverflow=off  RndMeth=Floor
  Data Type Conversion5 : DataTypeConversion  OutDataTypeStr=int8  SaturateOnIntegerOverflow=off  RndMeth=Floor
  Data Type Conversion8 : DataTypeConversion  OutDataTypeStr=boolean  SaturateOnIntegerOverflow=off  RndMeth=Floor
  CCAN_GW_MRR_FRObj_0x279FromOutData : Outport  OutDataTypeStr=Bus:CCAN_GW_MRR_FRObj_0x279
  wires:
  CAN FD Unpack/1 -> Data Type Conversion1/1
  CAN FD Unpack/2 -> Data Type Conversion2/1
  CAN FD Unpack/3 -> Data Type Conversion3/1
  CAN FD Unpack/4 -> Data Type Conversion4/1
  CAN FD Unpack/5 -> Data Type Conversion5/1
  CAN FD Unpack/6 -> Data Type Conversion6/1
  CAN FD Unpack/7 -> Data Type Conversion7/1
  CAN FD Unpack/8 -> Data Type Conversion8/1
  Data Type Conversion1/1 -> Bus Creator/1  "MRR_FFTargetDetection"
  Data Type Conversion2/1 -> Bus Creator/2  "MRR_FF_Obj_0x_class"
  Data Type Conversion3/1 -> Bus Creator/3  "MRR_FF_Object_dx"
  Data Type Conversion4/1 -> Bus Creator/4  "MRR_FF_Object_dy"
  Data Type Conversion5/1 -> Bus Creator/5  "MRR_F_Obj_0x_class"
  Data Type Conversion6/1 -> Bus Creator/6  "MRR_F_Object_dx"
  Data Type Conversion7/1 -> Bus Creator/7  "MRR_F_Object_dy"
  Data Type Conversion8/1 -> Bus Creator/8  "MRR_PedDetection"
  Bus Creator/1 -> CCAN_GW_MRR_FRObj_0x279FromOutData/1  "CCAN_GW_MRR_FRObj_0x279FromOutData"
  CCAN_GW_MRR_FRObj_0x279FromInData/1 -> CAN FD Unpack/1  "CCAN_GW_MRR_FRObj_0x279FromInData"

== system ALL_JP360_DBW_V6_5_1103/MsgFromCAN/CCAN_GW_MsgFromCAN/CCAN_GW_MRR_LRObj_0x480 ==
  CCAN_GW_MRR_LRObj_0x480FromInData : Inport  OutDataTypeStr=Bus:CAN_FD_MESSAGE_BUS
  Bus Creator : BusCreator  Inputs=8  OutDataTypeStr=Bus:CCAN_GW_MRR_LRObj_0x480  NonVirtualBus=on
  CAN FD Unpack : canfdmsglib/CAN FD Unpack  CANdbFile=HiFire_JPT360_CCAN_Matrix_CAN_V1.72_VP_ADCU.dbc  MsgList=(none)  MsgName=MRR_LRObj_0x480  ProtocolMode=CAN FD  MsgIDType=Standard (11-bit identifier)  MsgIdentifier=1152  MsgLength=8  SignalInfo={'MRR_L_Obj_0x_class','16','3','BE','unsigned','Standard','0','1','0','0','7';'MRR_L_Object_dx','12','12','BE','unsigned','Standard','0','0.0625','0','0','255.875';'MRR_L_Object_dy','19','9','BE','unsigned','Standard','0','0.0625','-15','-15','15';'MRR_LeftTargetDetection','54','1','BE','unsigned','Standard','0','1','0','0','1';'MRR_R_Obj_0x_class','40','3','BE','unsigned','Standard','0','1','0','0','7';'MRR_R_Object_dx','36','12','BE','unsigned','Standard','0','0.0625','0','0','255.875';'MRR_R_Object_dy','43','9','BE','unsigned','Standard','0','0.0625','-15','-15','15';'MRR_RightTargetDetection','55','1','BE','unsigned','Standard','0','1','0','0','1'}  IDPort=off  TimestampPort=off  ErrorPort=off  RemotePort=off  LengthPort=off  StatusPort=off  BRSPort=off  ESIPort=off  DLCPort=off  ApplyMinMax=off
      settings: SourceProductBaseCode=XP,ME,VN  DataFormat=CANdb specified signals
  Data Type Conversion1 : DataTypeConversion  OutDataTypeStr=int8  SaturateOnIntegerOverflow=off  RndMeth=Floor
  Data Type Conversion{2..3,6..7} (4 alike) : DataTypeConversion  OutDataTypeStr=single  SaturateOnIntegerOverflow=off  RndMeth=Floor
  Data Type Conversion4 : DataTypeConversion  OutDataTypeStr=boolean  SaturateOnIntegerOverflow=off  RndMeth=Floor
  Data Type Conversion5 : DataTypeConversion  OutDataTypeStr=int8  SaturateOnIntegerOverflow=off  RndMeth=Floor
  Data Type Conversion8 : DataTypeConversion  OutDataTypeStr=boolean  SaturateOnIntegerOverflow=off  RndMeth=Floor
  CCAN_GW_MRR_LRObj_0x480FromOutData : Outport  OutDataTypeStr=Bus:CCAN_GW_MRR_LRObj_0x480
  wires:
  CAN FD Unpack/1 -> Data Type Conversion1/1
  CAN FD Unpack/2 -> Data Type Conversion2/1
  CAN FD Unpack/3 -> Data Type Conversion3/1
  CAN FD Unpack/4 -> Data Type Conversion4/1
  CAN FD Unpack/5 -> Data Type Conversion5/1
  CAN FD Unpack/6 -> Data Type Conversion6/1
  CAN FD Unpack/7 -> Data Type Conversion7/1
  CAN FD Unpack/8 -> Data Type Conversion8/1
  Data Type Conversion1/1 -> Bus Creator/1  "MRR_L_Obj_0x_class"
  Data Type Conversion2/1 -> Bus Creator/2  "MRR_L_Object_dx"
  Data Type Conversion3/1 -> Bus Creator/3  "MRR_L_Object_dy"
  Data Type Conversion4/1 -> Bus Creator/4  "MRR_LeftTargetDetection"
  Data Type Conversion5/1 -> Bus Creator/5  "MRR_R_Obj_0x_class"
  Data Type Conversion6/1 -> Bus Creator/6  "MRR_R_Object_dx"
  Data Type Conversion7/1 -> Bus Creator/7  "MRR_R_Object_dy"
  Data Type Conversion8/1 -> Bus Creator/8  "MRR_RightTargetDetection"
  Bus Creator/1 -> CCAN_GW_MRR_LRObj_0x480FromOutData/1  "CCAN_GW_MRR_LRObj_0x480FromOutData"
  CCAN_GW_MRR_LRObj_0x480FromInData/1 -> CAN FD Unpack/1  "CCAN_GW_MRR_LRObj_0x480FromInData"

== system ALL_JP360_DBW_V6_5_1103/MsgFromCAN/CCAN_GW_MsgFromCAN/CCAN_GW_SAS_Sensor_0x175 ==
  CCAN_GW_SAS_Sensor_0x175FromInData : Inport  OutDataTypeStr=Bus:CAN_FD_MESSAGE_BUS
  Bus Creator : BusCreator  Inputs=10  OutDataTypeStr=Bus:CCAN_GW_SAS_Sensor_0x175  NonVirtualBus=on
  CAN FD Unpack : canfdmsglib/CAN FD Unpack  CANdbFile=HiFire_JPT360_CCAN_Matrix_CAN_V1.72_VP_ADCU.dbc  MsgList=(none)  MsgName=SAS_Sensor_0x175  ProtocolMode=CAN FD  MsgIDType=Standard (11-bit identifier)  MsgIdentifier=373  MsgLength=8  SignalInfo={'Checksum_0x175','56','8','BE','unsigned','Standard','0','1','0','0','255';'RollingCounter_0x175','48','4','BE','unsigned','Standard','0','1','0','0','15';'SAS_Raw_SASStsSnsr','54','1','BE','unsigned','Standard','0','1','0','0','1';'SAS_Raw_SteerWheelAngle','24','16','BE','unsigned','Standard','0','0.0238','-780','-780','779.7';'SAS_SASStsCal','53','1','BE','unsigned','Standard','0','1','0','0','1';'SAS_SASStsSnsr','55','1','BE','unsigned','Standard','0','1','0','0','1';'SAS_SteerWheelAngle','8','16','BE','unsigned','Standard','0','0.0238','-780','-780','779.7';'SAS_SteerWheelRotSpd','42','14','BE','unsigned','Standard','0','0.125','-1024','-1024','1023.75';'SAS_SteerWheelRotSpdStatus','41','1','BE','unsigned','Standard','0','1','0','0','1';'SAS_TrimmingSts','40','1','BE','unsigned','Standard','0','1','0','0','1'}  IDPort=off  TimestampPort=off  ErrorPort=off  RemotePort=off  LengthPort=off  StatusPort=off  BRSPort=off  ESIPort=off  DLCPort=off  ApplyMinMax=off
      settings: SourceProductBaseCode=XP,ME,VN  DataFormat=CANdb specified signals
  Data Type Conversion1 : DataTypeConversion  OutDataTypeStr=uint8  SaturateOnIntegerOverflow=off  RndMeth=Floor
  Data Type Conversion{3,5..6,9..10} (5 alike) : DataTypeConversion  OutDataTypeStr=boolean  SaturateOnIntegerOverflow=off  RndMeth=Floor
  Data Type Conversion2 : DataTypeConversion  OutDataTypeStr=int8  SaturateOnIntegerOverflow=off  RndMeth=Floor
  Data Type Conversion4 : DataTypeConversion  OutDataTypeStr=single  SaturateOnIntegerOverflow=off  RndMeth=Floor
  Data Type Conversion7 : DataTypeConversion  OutDataTypeStr=single  SaturateOnIntegerOverflow=off  RndMeth=Floor
  Data Type Conversion8 : DataTypeConversion  OutDataTypeStr=single  SaturateOnIntegerOverflow=off  RndMeth=Floor
  CCAN_GW_SAS_Sensor_0x175FromOutData : Outport  OutDataTypeStr=Bus:CCAN_GW_SAS_Sensor_0x175
  wires:
  CAN FD Unpack/1 -> Data Type Conversion1/1
  CAN FD Unpack/2 -> Data Type Conversion2/1
  CAN FD Unpack/3 -> Data Type Conversion3/1
  CAN FD Unpack/4 -> Data Type Conversion4/1
  CAN FD Unpack/5 -> Data Type Conversion5/1
  CAN FD Unpack/6 -> Data Type Conversion6/1
  CAN FD Unpack/7 -> Data Type Conversion7/1
  CAN FD Unpack/8 -> Data Type Conversion8/1
  CAN FD Unpack/9 -> Data Type Conversion9/1
  CAN FD Unpack/10 -> Data Type Conversion10/1
  Data Type Conversion1/1 -> Bus Creator/1  "Checksum_0x175"
  Data Type Conversion2/1 -> Bus Creator/2  "RollingCounter_0x175"
  Data Type Conversion3/1 -> Bus Creator/3  "SAS_Raw_SASStsSnsr"
  Data Type Conversion4/1 -> Bus Creator/4  "SAS_Raw_SteerWheelAngle"
  Data Type Conversion5/1 -> Bus Creator/5  "SAS_SASStsCal"
  Data Type Conversion6/1 -> Bus Creator/6  "SAS_SASStsSnsr"
  Data Type Conversion7/1 -> Bus Creator/7  "SAS_SteerWheelAngle"
  Data Type Conversion8/1 -> Bus Creator/8  "SAS_SteerWheelRotSpd"
  Data Type Conversion9/1 -> Bus Creator/9  "SAS_SteerWheelRotSpdStatus"
  Data Type Conversion10/1 -> Bus Creator/10  "SAS_TrimmingSts"
  Bus Creator/1 -> CCAN_GW_SAS_Sensor_0x175FromOutData/1  "CCAN_GW_SAS_Sensor_0x175FromOutData"
  CCAN_GW_SAS_Sensor_0x175FromInData/1 -> CAN FD Unpack/1  "CCAN_GW_SAS_Sensor_0x175FromInData"
